simulink model "Microgrid_transition_model_111821_ben"  (R2020a)
settings: Solver=VariableStepAuto  StartTime=0.0  StopTime=16  MaxStep=1e-4  RelTol=1e-3
PreLoadFcn:
  | %run('FC_microgrid_param.m')
  | %load('gen_grid_init.mat')
InitFcn:
  | %load myisoModel_init;
  | run('FC_microgrid_param.m')
  | tic
  | run('CARTinitFcn.m')
  | %caseNo = 2;
  | 
  | %if (caseNo == 1)
  | %set_param(['Isolated_grid_paper_model_022521/SignalGen'], 'ActiveScenario', 'PStep222kW');
  | %else
  | %set_param(['Isolated_grid_paper_model_022521/SignalGen'], 'ActiveScenario', 'QStep222kVAr');
  | 
  | %end;
StopFcn:
  | toc
undefined symbols (not defined in the file): breakpoints1, breakpoints2, cc_kp, cp_table_data, ctrl, D1, Delta, DiscIntNeverNeededParam, DT, FC_BESS, FC_PV_FirstSolar, find_system, gcbh, libFC_BESS, libFC_PV, LowerLimit, magnitude, oversize, pll_ki, pll_kp, pq_ts, sps_rtmsupport, timer, Ts, ts, Ts_APC, Ts_Control, Ts_Power, UpperLimit
libraries: powerlib x152, powerlib_extras x100, simulink x95, powerlib_meascontrol x86, eePowerMeasurement x26, pi_ctrl x16, simulink_extras x12, sps_avr x7, spsDieselMotorModel x3, libFSArray x2, SignalEditorBlockLib x2, libLgBattery x1
(part 6 of 14)

== system Microgrid_transition_model_111821_ben/../Control/Speed & Pitch Control ==
  note: Current Regulator
  note: IL ref
  note: Note :
      | This control system is based on the report:
      | Dynamic Modeling of GE 1.5 and 3.6 Wind Turbine-Generators;
      | Prepared by: Nicholas W. Miller, William W. Price, Juan J. Sanchez-Gasca;
      | October 27, 2003, Version 3.0
      | GE-Power Systems Energy Consulting
      | Copyright 2002 General Electric Company, U.S.A.
      |
      | Another reference is:
      |
      | DYNAMIC MODELING OF GE 1.5 AND 3.6 MW WIND TURBINE GENERATORS
      | FOR STABILITY SIMULATIONS
      | Nicholas W. Miller, Juan J. Sanchez-Gasca, William W. Price Robert W. Delmerico
      | GE Power Systems GE Research
      | Schenectady, NY Niskayuna, NY
      |
      | 0-7803-7989-6/03/$17.00 02003 IEEE
  note: Speed Regulator
  note: Pitch Compensation
  note: Pitch Control
  wr : Inport
  Pmeas : Inport  Port=2
  IL : Inport  Port=3
  0-inf : Saturate  UpperLimit=inf  LowerLimit=0
  0-pitch_max : Saturate  UpperLimit=pitch_max  LowerLimit=0
  "0-pitch_max " : Saturate  UpperLimit=pitch_max  LowerLimit=0
  Constant2 : Constant
  Discrete PI Controller : Subsystem  DialogController=POWERSYS.PowerSysDialog  mask(Discrete PI Controller){Kp=Kp_speed, Ki=Ki_speed, Par_Limits=[1.1 0], Init=0, Ts=Ts}
      mask prompts: Kp "Proportional gain (Kp):"; Ki "Integral gain (Ki):"; Par_Limits "Output limits: [ Upper   Lower ]"; Init "Output initial value:"; Ts "Sample time:"
      mask help: This block implements a discrete PI controller.
      mask init:
      | UpperLimit=Par_Limits(1);
      | LowerLimit=Par_Limits(2);
      | power_initmask();
      mask Help: This block is part of a subset of blocks in the Extras library that does not have documentation associated with it, other than the block mask description.
      mask Display: disp('PI');
  Discrete PI Controller1 : Subsystem  DialogController=POWERSYS.PowerSysDialog  mask(Discrete PI Controller){Kp=Kp_compensation, Ki=Ki_compensation, Par_Limits=[pitch_max 0], Init=0, Ts=Ts}
      mask prompts: Kp "Proportional gain (Kp):"; Ki "Integral gain (Ki):"; Par_Limits "Output limits: [ Upper   Lower ]"; Init "Output initial value:"; Ts "Sample time:"
      mask help: This block implements a discrete PI controller.
      mask init:
      | UpperLimit=Par_Limits(1);
      | LowerLimit=Par_Limits(2);
      | power_initmask();
      mask Help: This block is part of a subset of blocks in the Extras library that does not have documentation associated with it, other than the block mask description.
      mask Display: disp('PI');
  Discrete PI Controller2 : Subsystem  DialogController=POWERSYS.PowerSysDialog  mask(Discrete PI Controller){Kp=Kp_boost_cur_reg, Ki=Ki_boost_cur_reg, Par_Limits=[1 0], Init=0.5, Ts=Ts}
      mask prompts: Kp "Proportional gain (Kp):"; Ki "Integral gain (Ki):"; Par_Limits "Output limits: [ Upper   Lower ]"; Init "Output initial value:"; Ts "Sample time:"
      mask help: This block implements a discrete PI controller.
      mask init:
      | UpperLimit=Par_Limits(1);
      | LowerLimit=Par_Limits(2);
      | power_initmask();
      mask Help: This block is part of a subset of blocks in the Extras library that does not have documentation associated with it, other than the block mask description.
      mask Display: disp('PI');
  First-Order Filter : powerlib_meascontrol/Filters/First-Order Filter  FilterType=Lowpass  Tc=Pitch_time_constant  Ts=Ts  Initialize=on  Vac_Init=[0.8 -25 60]*0  Vdc_Init=0  PlotResponse=off  FreqRange="[0,  200,  1]"
      settings: SourceProductBaseCode=MT,PS
  First-Order Filter1 : powerlib_meascontrol/Filters/First-Order Filter  FilterType=Lowpass  Tc=T_speed  Ts=Ts  Initialize=on  Vac_Init=[0, 0, 0]  Vdc_Init=1+init(1)/100  PlotResponse=off  FreqRange="[0,  200,  1]"
      settings: SourceProductBaseCode=MT,PS
  Gain2 : Gain  Gain=Kp_pitch  SaturateOnIntegerOverflow=on  OutDataTypeStr=Inherit: Same as input  ParamDataTypeStr=Inherit: Same as input
  Rate Limiter   1 : RateLimiter  RisingSlewLimit=pitch_rate  FallingSlewLimit=-pitch_rate
  Sum : Sum  Inputs=-+  SaturateOnIntegerOverflow=on
  Sum1 : Sum  Inputs=|+-
  Sum2 : Sum  Inputs=|+-  SaturateOnIntegerOverflow=on
  Sum3 : Sum  Inputs=|++
  Sum4 : Sum  Inputs=|+-
  Switch : Switch  Threshold=0.75
  Tracking Curve : Fcn  Expr=-0.5551*u(1)^2+1.183*u(1)+0.425
  pu_elec->pu_mec : Gain  Gain=Pnom/Pmec
  wref : Constant
  Duty_Cycle : Outport  VectorParamsAs1DForOutWhenUnconnected=off
  Pitch (deg) : Outport  Port=2  VectorParamsAs1DForOutWhenUnconnected=off
  wires:
  Discrete PI Controller2/1(Out) -> Duty_Cycle/1  "Duty cycle"
  IL/1 -> Sum4/2
  Sum4/1 -> Discrete PI Controller2/1(Error)
  Discrete PI Controller/1(Out) -> Sum4/1
  Tracking Curve/1 -> Switch/3
  First-Order Filter1/1 -> Sum/1, Sum1/2  "wref"
  Sum2/1 -> Discrete PI Controller1/1(Error)
  First-Order Filter/1 -> Pitch (deg)/1  "Pitch"
  Sum/1 -> Gain2/1
  "0-pitch_max "/1 -> First-Order Filter/1
  0-pitch_max/1 -> Sum3/1  "Pitch_contrl"
  Pmeas/1 -> 0-inf/1
  Discrete PI Controller1/1(Out) -> Sum3/2  "Pitch_comp"
  Gain2/1 -> 0-pitch_max/1
  Rate Limiter   1/1 -> "0-pitch_max "/1
  Sum3/1 -> Rate Limiter   1/1
  Constant2/1 -> Sum2/2  "Pref"
  Sum1/1 -> Discrete PI Controller/1(Error)
  Switch/1 -> First-Order Filter1/1
  wref/1 -> Switch/1
  pu_elec->pu_mec/1 -> Switch/2, Sum2/1, Tracking Curve/1  "Pmes"
  0-inf/1 -> pu_elec->pu_mec/1
  wr/1 -> Sum1/1, Sum/2  "wr"

== system Microgrid_transition_model_111821_ben/Defferable Load (0-446.25 kW)/Switches/Switches ABC0 ==
  P_ABC : Inport
  Demux : Demux  Outputs=3
      settings: DisplayOption=none
  Switch A : powerlib/Power Electronics/Ideal Switch  Ron=Ron_switch  Lon=0  IC=Status(1)  Rs=Rs_snubber  Cs=Cs_snubber  Measurements=off
      settings: AttributesFormatString=\n  SourceProductBaseCode=MT,PS
  Switch B : powerlib/Power Electronics/Ideal Switch  Ron=Ron_switch  Lon=0  IC=Status(1)  Rs=Rs_snubber  Cs=Cs_snubber  Measurements=off
      settings: AttributesFormatString=\n  SourceProductBaseCode=MT,PS
  Switch C : powerlib/Power Electronics/Ideal Switch  Ron=Ron_switch  Lon=0  IC=Status(1)  Rs=Rs_snubber  Cs=Cs_snubber  Measurements=off
      settings: AttributesFormatString=\n  SourceProductBaseCode=MT,PS
  A : PMIOPort  Side=Left
  B : PMIOPort  Port=2  Side=Left
  C : PMIOPort  Port=3  Side=Left
  "A " : PMIOPort  Port=4  Side=Right
  "B " : PMIOPort  Port=5  Side=Right
  "C " : PMIOPort  Port=6  Side=Right
  wires:
  P_ABC/1 -> Demux/1
  Demux/3 -> Switch C/1
  Demux/2 -> Switch B/1
  Demux/1 -> Switch A/1
  connections:
  Switch C/RConn1 -- "C "/RConn1
  Switch B/RConn1 -- "B "/RConn1
  Switch A/RConn1 -- "A "/RConn1
  C/RConn1 -- Switch C/LConn1
  B/RConn1 -- Switch B/LConn1
  A/RConn1 -- Switch A/LConn1

== system Microgrid_transition_model_111821_ben/Defferable Load (0-446.25 kW)/Switches/Switches ABC1 ==
  P_ABC : Inport
  Demux : Demux  Outputs=3
      settings: DisplayOption=none
  Switch A : powerlib/Power Electronics/Ideal Switch  Ron=Ron_switch  Lon=0  IC=Status(2)  Rs=Rs_snubber  Cs=Cs_snubber  Measurements=off
      settings: AttributesFormatString=\n  SourceProductBaseCode=MT,PS
  Switch B : powerlib/Power Electronics/Ideal Switch  Ron=Ron_switch  Lon=0  IC=Status(2)  Rs=Rs_snubber  Cs=Cs_snubber  Measurements=off
      settings: AttributesFormatString=\n  SourceProductBaseCode=MT,PS
  Switch C : powerlib/Power Electronics/Ideal Switch  Ron=Ron_switch  Lon=0  IC=Status(2)  Rs=Rs_snubber  Cs=Cs_snubber  Measurements=off
      settings: AttributesFormatString=\n  SourceProductBaseCode=MT,PS
  A : PMIOPort  Side=Left
  B : PMIOPort  Port=2  Side=Left
  C : PMIOPort  Port=3  Side=Left
  "A " : PMIOPort  Port=4  Side=Right
  "B " : PMIOPort  Port=5  Side=Right
  "C " : PMIOPort  Port=6  Side=Right
  wires:
  Demux/1 -> Switch A/1
  Demux/2 -> Switch B/1
  Demux/3 -> Switch C/1
  P_ABC/1 -> Demux/1
  connections:
  A/RConn1 -- Switch A/LConn1
  B/RConn1 -- Switch B/LConn1
  Switch A/RConn1 -- "A "/RConn1
  Switch B/RConn1 -- "B "/RConn1
  Switch C/RConn1 -- "C "/RConn1
  C/RConn1 -- Switch C/LConn1

== system Microgrid_transition_model_111821_ben/Defferable Load (0-446.25 kW)/Switches/Switches ABC2 ==
  P_ABC : Inport
  Demux : Demux  Outputs=3
      settings: DisplayOption=none
  Switch A : powerlib/Power Electronics/Ideal Switch  Ron=Ron_switch  Lon=0  IC=Status(3)  Rs=Rs_snubber  Cs=Cs_snubber  Measurements=off
      settings: AttributesFormatString=\n  SourceProductBaseCode=MT,PS
  Switch B : powerlib/Power Electronics/Ideal Switch  Ron=Ron_switch  Lon=0  IC=Status(3)  Rs=Rs_snubber  Cs=Cs_snubber  Measurements=off
      settings: AttributesFormatString=\n  SourceProductBaseCode=MT,PS
  Switch C : powerlib/Power Electronics/Ideal Switch  Ron=Ron_switch  Lon=0  IC=Status(3)  Rs=Rs_snubber  Cs=Cs_snubber  Measurements=off
      settings: AttributesFormatString=\n  SourceProductBaseCode=MT,PS
  A : PMIOPort  Side=Left
  B : PMIOPort  Port=2  Side=Left
  C : PMIOPort  Port=3  Side=Left
  "A " : PMIOPort  Port=4  Side=Right
  "B " : PMIOPort  Port=5  Side=Right
  "C " : PMIOPort  Port=6  Side=Right
  wires:
  P_ABC/1 -> Demux/1
  Demux/3 -> Switch C/1
  Demux/2 -> Switch B/1
  Demux/1 -> Switch A/1
  connections:
  Switch C/RConn1 -- "C "/RConn1
  Switch B/RConn1 -- "B "/RConn1
  Switch A/RConn1 -- "A "/RConn1
  A/RConn1 -- Switch A/LConn1
  B/RConn1 -- Switch B/LConn1
  C/RConn1 -- Switch C/LConn1

== system Microgrid_transition_model_111821_ben/Defferable Load (0-446.25 kW)/Switches/Switches ABC3 ==
  P_ABC : Inport
  Demux : Demux  Outputs=3
      settings: DisplayOption=none
  Switch A : powerlib/Power Electronics/Ideal Switch  Ron=Ron_switch  Lon=0  IC=Status(4)  Rs=Rs_snubber  Cs=Cs_snubber  Measurements=off
      settings: AttributesFormatString=\n  SourceProductBaseCode=MT,PS
  Switch B : powerlib/Power Electronics/Ideal Switch  Ron=Ron_switch  Lon=0  IC=Status(4)  Rs=Rs_snubber  Cs=Cs_snubber  Measurements=off
      settings: AttributesFormatString=\n  SourceProductBaseCode=MT,PS
  Switch C : powerlib/Power Electronics/Ideal Switch  Ron=Ron_switch  Lon=0  IC=Status(4)  Rs=Rs_snubber  Cs=Cs_snubber  Measurements=off
      settings: AttributesFormatString=\n  SourceProductBaseCode=MT,PS
  A : PMIOPort  Side=Left
  B : PMIOPort  Port=2  Side=Left
  C : PMIOPort  Port=3  Side=Left
  "A " : PMIOPort  Port=4  Side=Right
  "B " : PMIOPort  Port=5  Side=Right
  "C " : PMIOPort  Port=6  Side=Right
  wires:
  Demux/1 -> Switch A/1
  Demux/2 -> Switch B/1
  Demux/3 -> Switch C/1
  P_ABC/1 -> Demux/1
  connections:
  C/RConn1 -- Switch C/LConn1
  B/RConn1 -- Switch B/LConn1
  A/RConn1 -- Switch A/LConn1
  Switch A/RConn1 -- "A "/RConn1
  Switch B/RConn1 -- "B "/RConn1
  Switch C/RConn1 -- "C "/RConn1

== system Microgrid_transition_model_111821_ben/Defferable Load (0-446.25 kW)/Switches/Switches ABC4 ==
  P_ABC : Inport
  Demux : Demux  Outputs=3
      settings: DisplayOption=none
  Switch A : powerlib/Power Electronics/Ideal Switch  Ron=Ron_switch  Lon=0  IC=Status(5)  Rs=Rs_snubber  Cs=Cs_snubber  Measurements=off
      settings: AttributesFormatString=\n  SourceProductBaseCode=MT,PS
  Switch B : powerlib/Power Electronics/Ideal Switch  Ron=Ron_switch  Lon=0  IC=Status(5)  Rs=Rs_snubber  Cs=Cs_snubber  Measurements=off
      settings: AttributesFormatString=\n  SourceProductBaseCode=MT,PS
  Switch C : powerlib/Power Electronics/Ideal Switch  Ron=Ron_switch  Lon=0  IC=Status(5)  Rs=Rs_snubber  Cs=Cs_snubber  Measurements=off
      settings: AttributesFormatString=\n  SourceProductBaseCode=MT,PS
  A : PMIOPort  Side=Left
  B : PMIOPort  Port=2  Side=Left
  C : PMIOPort  Port=3  Side=Left
  "A " : PMIOPort  Port=4  Side=Right
  "B " : PMIOPort  Port=5  Side=Right
  "C " : PMIOPort  Port=6  Side=Right
  wires:
  P_ABC/1 -> Demux/1
  Demux/3 -> Switch C/1
  Demux/2 -> Switch B/1
  Demux/1 -> Switch A/1
  connections:
  Switch C/RConn1 -- "C "/RConn1
  Switch B/RConn1 -- "B "/RConn1
  Switch A/RConn1 -- "A "/RConn1
  A/RConn1 -- Switch A/LConn1
  B/RConn1 -- Switch B/LConn1
  C/RConn1 -- Switch C/LConn1

== system Microgrid_transition_model_111821_ben/Defferable Load (0-446.25 kW)/Switches/Switches ABC5 ==
  P_ABC : Inport
  Demux : Demux  Outputs=3
      settings: DisplayOption=none
  Switch A : powerlib/Power Electronics/Ideal Switch  Ron=Ron_switch  Lon=0  IC=Status(6)  Rs=Rs_snubber  Cs=Cs_snubber  Measurements=off
      settings: AttributesFormatString=\n  SourceProductBaseCode=MT,PS
  Switch B : powerlib/Power Electronics/Ideal Switch  Ron=Ron_switch  Lon=0  IC=Status(6)  Rs=Rs_snubber  Cs=Cs_snubber  Measurements=off
      settings: AttributesFormatString=\n  SourceProductBaseCode=MT,PS
  Switch C : powerlib/Power Electronics/Ideal Switch  Ron=Ron_switch  Lon=0  IC=Status(6)  Rs=Rs_snubber  Cs=Cs_snubber  Measurements=off
      settings: AttributesFormatString=\n  SourceProductBaseCode=MT,PS
  A : PMIOPort  Side=Left
  B : PMIOPort  Port=2  Side=Left
  C : PMIOPort  Port=3  Side=Left
  "A " : PMIOPort  Port=4  Side=Right
  "B " : PMIOPort  Port=5  Side=Right
  "C " : PMIOPort  Port=6  Side=Right
  wires:
  Demux/1 -> Switch A/1
  Demux/2 -> Switch B/1
  Demux/3 -> Switch C/1
  P_ABC/1 -> Demux/1
  connections:
  C/RConn1 -- Switch C/LConn1
  B/RConn1 -- Switch B/LConn1
  A/RConn1 -- Switch A/LConn1
  Switch A/RConn1 -- "A "/RConn1
  Switch B/RConn1 -- "B "/RConn1
  Switch C/RConn1 -- "C "/RConn1

== system Microgrid_transition_model_111821_ben/Defferable Load (0-446.25 kW)/Switches/Switches ABC6 ==
  P_ABC : Inport
  Demux : Demux  Outputs=3
      settings: DisplayOption=none
  Switch A : powerlib/Power Electronics/Ideal Switch  Ron=Ron_switch  Lon=0  IC=Status(7)  Rs=Rs_snubber  Cs=Cs_snubber  Measurements=off
      settings: AttributesFormatString=\n  SourceProductBaseCode=MT,PS
  Switch B : powerlib/Power Electronics/Ideal Switch  Ron=Ron_switch  Lon=0  IC=Status(7)  Rs=Rs_snubber  Cs=Cs_snubber  Measurements=off
      settings: AttributesFormatString=\n  SourceProductBaseCode=MT,PS
  Switch C : powerlib/Power Electronics/Ideal Switch  Ron=Ron_switch  Lon=0  IC=Status(7)  Rs=Rs_snubber  Cs=Cs_snubber  Measurements=off
      settings: AttributesFormatString=\n  SourceProductBaseCode=MT,PS
  A : PMIOPort  Side=Left
  B : PMIOPort  Port=2  Side=Left
  C : PMIOPort  Port=3  Side=Left
  "A " : PMIOPort  Port=4  Side=Right
  "B " : PMIOPort  Port=5  Side=Right
  "C " : PMIOPort  Port=6  Side=Right
  wires:
  P_ABC/1 -> Demux/1
  Demux/3 -> Switch C/1
  Demux/2 -> Switch B/1
  Demux/1 -> Switch A/1
  connections:
  Switch C/RConn1 -- "C "/RConn1
  Switch B/RConn1 -- "B "/RConn1
  Switch A/RConn1 -- "A "/RConn1
  A/RConn1 -- Switch A/LConn1
  B/RConn1 -- Switch B/LConn1
  C/RConn1 -- Switch C/LConn1

== system Microgrid_transition_model_111821_ben/Defferable Load (0-446.25 kW)/Switches/Switches ABC7 ==
  P_ABC : Inport
  Demux : Demux  Outputs=3
      settings: DisplayOption=none
  Switch A : powerlib/Power Electronics/Ideal Switch  Ron=Ron_switch  Lon=0  IC=Status(8)  Rs=Rs_snubber  Cs=Cs_snubber  Measurements=off
      settings: AttributesFormatString=\n  SourceProductBaseCode=MT,PS
  Switch B : powerlib/Power Electronics/Ideal Switch  Ron=Ron_switch  Lon=0  IC=Status(8)  Rs=Rs_snubber  Cs=Cs_snubber  Measurements=off
      settings: AttributesFormatString=\n  SourceProductBaseCode=MT,PS
  Switch C : powerlib/Power Electronics/Ideal Switch  Ron=Ron_switch  Lon=0  IC=Status(8)  Rs=Rs_snubber  Cs=Cs_snubber  Measurements=off
      settings: AttributesFormatString=\n  SourceProductBaseCode=MT,PS
  A : PMIOPort  Side=Left
  B : PMIOPort  Port=2  Side=Left
  C : PMIOPort  Port=3  Side=Left
  "A " : PMIOPort  Port=4  Side=Right
  "B " : PMIOPort  Port=5  Side=Right
  "C " : PMIOPort  Port=6  Side=Right
  wires:
  Demux/1 -> Switch A/1
  Demux/2 -> Switch B/1
  Demux/3 -> Switch C/1
  P_ABC/1 -> Demux/1
  connections:
  C/RConn1 -- Switch C/LConn1
  B/RConn1 -- Switch B/LConn1
  A/RConn1 -- Switch A/LConn1
  Switch A/RConn1 -- "A "/RConn1
  Switch B/RConn1 -- "B "/RConn1
  Switch C/RConn1 -- "C "/RConn1

== system Microgrid_transition_model_111821_ben/FC_BESS/SMAInverter/85_SMAControl ==
  Uabc : Inport
  Uabc_inv : Inport  Port=2
  Iabc : Inport  Port=3
  CB_status : Inport  Port=4
  Control : Inport  Port=5
  Bus Creator1 : BusCreator  Inputs=2
  Bus Creator5 : BusCreator  Inputs=1
  Bus Selector : BusSelector  OutputSignals=p_ref,q_ref,f_ref,v_ref,GF_mode
  InvControl : Subsystem  mask{Ts=Ts_Control, Unpp=400, Pn=1e6}
      mask prompts: Ts "Control sample time [s]"; Unpp "Nominal AC voltage [Vpp]"; Pn "Nominal Power [W]"
      mask init:
      | Unom = Unpp / sqrt(3);
      | Inom = Pn/3/Unom;
  Rate Transition{,1..2,4..7,9..10} (9 alike) : RateTransition  Integrity=off  OutPortSampleTime=Ts_Control
  Rate Transition3 : RateTransition  OutPortSampleTime=Ts
  Rate Transition8 : RateTransition  OutPortSampleTime=Ts
  Scope : Scope
  Step : Step  Time=3  Before=1  After=0  SampleTime=Ts
  Step1 : Step  Time=6.4  SampleTime=Ts
  Sum : Sum  Inputs=|++
  CtrlOut : Outport
  wires:
  Rate Transition4/1 -> InvControl/5(pref)
  Iabc/1 -> Rate Transition1/1
  Rate Transition2/1 -> InvControl/4(cb_stat)
  Rate Transition1/1 -> InvControl/3(Iabc)
  Rate Transition/1 -> InvControl/1(Uabc)
  Rate Transition8/1 -> Bus Creator5/1  "Close"
  Step/1 -> Sum/1
  InvControl/1(Uabc_ref) -> Rate Transition3/1
  Rate Transition3/1 -> Bus Creator1/1  "Uabc"
  Uabc/1 -> Rate Transition/1
  CB_status/1 -> Rate Transition2/1
  Bus Creator5/1 -> Bus Creator1/2  "ToCB"
  Bus Creator1/1 -> CtrlOut/1
  Bus Selector/1 -> Rate Transition4/1  "<p_ref>"
  Bus Selector/2 -> Rate Transition5/1  "<q_ref>"
  Bus Selector/3 -> Rate Transition6/1  "<f_ref>"
  Bus Selector/4 -> Rate Transition7/1  "<v_ref>"
  Bus Selector/5 -> Rate Transition9/1  "<GF_mode>"
  Rate Transition9/1 -> InvControl/9(GF_mode_en)
  Rate Transition7/1 -> InvControl/8(vref)
  Rate Transition5/1 -> InvControl/6(qref)
  Rate Transition6/1 -> InvControl/7(fref)
  Control/1 -> Bus Selector/1
  Uabc_inv/1 -> Rate Transition10/1
  Rate Transition10/1 -> InvControl/2(Uabc_inv)
  Step1/1 -> Sum/2
  Sum/1 -> Scope/1, Rate Transition8/1

== system Microgrid_transition_model_111821_ben/FC_BESS/SMAInverter/BESS Inverter ==
  ctrl : Inport
  Controlled Voltage Source : powerlib/Electrical Sources/Controlled Voltage Source  Initialize=on  Source_Type=AC  Amplitude=0  Phase=0  Frequency=0  Measurements=None
  Controlled Voltage Source1 : powerlib/Electrical Sources/Controlled Voltage Source  Initialize=on  Source_Type=AC  Amplitude=0  Phase=0  Frequency=0  Measurements=None
  Controlled Voltage Source2 : powerlib/Electrical Sources/Controlled Voltage Source  Initialize=on  Source_Type=AC  Amplitude=0  Phase=0  Frequency=0  Measurements=None
  Demux : Demux  Outputs=3
  A : PMIOPort  Side=Right
  N : PMIOPort  Port=2  Side=Left
  B : PMIOPort  Port=3  Side=Right
  C : PMIOPort  Port=4  Side=Right
  wires:
  ctrl/1 -> Demux/1
  Demux/3 -> Controlled Voltage Source2/1
  Demux/2 -> Controlled Voltage Source1/1
  Demux/1 -> Controlled Voltage Source/1
  connections:
  Controlled Voltage Source2/RConn1 -- C/RConn1
  Controlled Voltage Source1/RConn1 -- B/RConn1
  N/RConn1 -- Controlled Voltage Source1/LConn1 -- Controlled Voltage Source/LConn1 -- Controlled Voltage Source2/LConn1
  A/RConn1 -- Controlled Voltage Source/RConn1

== system Microgrid_transition_model_111821_ben/FC_BESS/SMAInverter/Subsystem ==
  GRI1 : powerlib/Measurements/Three-Phase V-I Measurement  VoltageMeasurement=phase-to-ground  SetLabelV=off  LabelV=Ugri  Vpu=off  VpuLL=off  CurrentMeasurement=yes  SetLabelI=off  LabelI=Igri  Ipu=off  Pbase=100e6  Vbase=500e3  OutputType=Complex  PhasorSimulation=off  PSBequivalent=0
  A : PMIOPort  Side=Left
  B : PMIOPort  Port=2  Side=Left
  a : PMIOPort  Port=3  Side=Right
  b : PMIOPort  Port=4  Side=Right
  C : PMIOPort  Port=5  Side=Left
  c : PMIOPort  Port=6  Side=Right
  tag scope: Igri=scoped, Ugri=scoped
  wires:
  GRI1/2 -> [Igri]
  GRI1/1 -> [Ugri]
  connections:
  GRI1/RConn1 -- a/RConn1
  GRI1/LConn1 -- A/RConn1
  GRI1/RConn2 -- b/RConn1
  GRI1/RConn3 -- c/RConn1
  GRI1/LConn2 -- B/RConn1
  GRI1/LConn3 -- C/RConn1

== system Microgrid_transition_model_111821_ben/FC_BESS/SMAInverter/Subsystem1 ==
  SmaINV : powerlib/Measurements/Three-Phase V-I Measurement  VoltageMeasurement=phase-to-ground  SetLabelV=off  LabelV=circuit_Usmainv  Vpu=off  VpuLL=off  CurrentMeasurement=yes  SetLabelI=off  LabelI=circuit_Ismainv  Ipu=off  Pbase=100e6  Vbase=500e3  OutputType=Complex  PhasorSimulation=off  PSBequivalent=0
  A : PMIOPort  Side=Left
  a : PMIOPort  Port=2  Side=Right
  B : PMIOPort  Port=3  Side=Left
  b : PMIOPort  Port=4  Side=Right
  C : PMIOPort  Port=5  Side=Left
  c : PMIOPort  Port=6  Side=Right
  tag scope: Iinv=scoped, Uinv=scoped
  wires:
  SmaINV/1 -> [Uinv]
  SmaINV/2 -> [Iinv]
  connections:
  SmaINV/RConn1 -- a/RConn1
  C/RConn1 -- SmaINV/LConn3
  SmaINV/LConn2 -- B/RConn1
  SmaINV/RConn2 -- b/RConn1
  SmaINV/RConn3 -- c/RConn1
  A/RConn1 -- SmaINV/LConn1

== system Microgrid_transition_model_111821_ben/FC_PV_FirstSolar/AllStringInverters/BESS Inverter ==
  ctrl : Inport
  Controlled Voltage Source : powerlib/Electrical Sources/Controlled Voltage Source  Initialize=on  Source_Type=AC  Amplitude=0  Phase=0  Frequency=0  Measurements=None
  Controlled Voltage Source1 : powerlib/Electrical Sources/Controlled Voltage Source  Initialize=on  Source_Type=AC  Amplitude=0  Phase=0  Frequency=0  Measurements=None
  Controlled Voltage Source2 : powerlib/Electrical Sources/Controlled Voltage Source  Initialize=on  Source_Type=AC  Amplitude=0  Phase=0  Frequency=0  Measurements=None
  Demux : Demux  Outputs=3
  A : PMIOPort  Side=Right
  N : PMIOPort  Port=2  Side=Left
  B : PMIOPort  Port=3  Side=Right
  C : PMIOPort  Port=4  Side=Right
  wires:
  Demux/1 -> Controlled Voltage Source/1
  Demux/2 -> Controlled Voltage Source1/1
  Demux/3 -> Controlled Voltage Source2/1
  ctrl/1 -> Demux/1
  connections:
  A/RConn1 -- Controlled Voltage Source/RConn1
  Controlled Voltage Source2/LConn1 -- Controlled Voltage Source/LConn1 -- Controlled Voltage Source1/LConn1 -- N/RConn1
  Controlled Voltage Source1/RConn1 -- B/RConn1
  Controlled Voltage Source2/RConn1 -- C/RConn1

== system Microgrid_transition_model_111821_ben/FC_PV_FirstSolar/AllStringInverters/PV_Control ==
  Uabc : Inport
  Uabc_inv : Inport  Port=2
  Iabc : Inport  Port=3
  CB_status : Inport  Port=4
  Control : Inport  Port=5
  Ppv : Inport  Port=6
  Bus Creator1 : BusCreator  Inputs=2
  Bus Creator5 : BusCreator  Inputs=1
  Bus Selector : BusSelector  OutputSignals=p_ref,q_ref,f_ref,v_ref,GF_mode
  InvControl : Subsystem  mask{Ts=Ts_Control, Unpp=600, Pn=430e3}
      mask prompts: Ts "Control sample time [s]"; Unpp "Nominal AC voltage [Vpp]"; Pn "Nominal Power [W]"
      mask init:
      | Unom = Unpp / sqrt(3);
      | Inom = Pn/3/Unom;
  Min : MinMax  Inputs=2
  Rate Transition{,1..2,4..7,9..10} (9 alike) : RateTransition  Integrity=off  OutPortSampleTime=Ts_Control
  Rate Transition3 : RateTransition  OutPortSampleTime=Ts
  Rate Transition8 : RateTransition  OutPortSampleTime=Ts
  Step : Step  Time=0.5  SampleTime=0
  Step1 : Step  Time=99  After=-1  SampleTime=0
  Sum : Sum  Inputs=|++
  CtrlOut : Outport
  wires:
  Rate Transition10/1 -> InvControl/2(Uabc_inv)
  Uabc_inv/1 -> Rate Transition10/1
  Control/1 -> Bus Selector/1
  Rate Transition6/1 -> InvControl/7(fref)
  Rate Transition5/1 -> InvControl/6(qref)
  Rate Transition7/1 -> InvControl/8(vref)
  Rate Transition9/1 -> InvControl/9(GF_mode_en)
  Bus Selector/5 -> Rate Transition9/1  "<GF_mode>"
  Bus Selector/4 -> Rate Transition7/1  "<v_ref>"
  Bus Selector/3 -> Rate Transition6/1  "<f_ref>"
  Bus Selector/2 -> Rate Transition5/1  "<q_ref>"
  Bus Selector/1 -> Min/1  "<p_ref>"
  Bus Creator1/1 -> CtrlOut/1
  Bus Creator5/1 -> Bus Creator1/2  "ToCB"
  CB_status/1 -> Rate Transition2/1
  Uabc/1 -> Rate Transition/1
  Rate Transition3/1 -> Bus Creator1/1  "Uabc"
  InvControl/1(Uabc_ref) -> Rate Transition3/1
  Step/1 -> Sum/1
  Rate Transition8/1 -> Bus Creator5/1  "Close"
  Rate Transition/1 -> InvControl/1(Uabc)
  Rate Transition1/1 -> InvControl/3(Iabc)
  Rate Transition2/1 -> InvControl/4(cb_stat)
  Iabc/1 -> Rate Transition1/1
  Rate Transition4/1 -> InvControl/5(pref)
  Ppv/1 -> Min/2
  Min/1 -> Rate Transition4/1
  Step1/1 -> Sum/2
  Sum/1 -> Rate Transition8/1

== system Microgrid_transition_model_111821_ben/FC_PV_FirstSolar/AllStringInverters/Subsystem1 ==
  SmaINV : powerlib/Measurements/Three-Phase V-I Measurement  VoltageMeasurement=phase-to-ground  SetLabelV=off  LabelV=circuit_Usmainv  Vpu=off  VpuLL=off  CurrentMeasurement=yes  SetLabelI=off  LabelI=circuit_Ismainv  Ipu=off  Pbase=100e6  Vbase=500e3  OutputType=Complex  PhasorSimulation=off  PSBequivalent=0
  A : PMIOPort  Side=Left
  a : PMIOPort  Port=2  Side=Right
  B : PMIOPort  Port=3  Side=Left
  b : PMIOPort  Port=4  Side=Right
  C : PMIOPort  Port=5  Side=Left
  c : PMIOPort  Port=6  Side=Right
  tag scope: Iinv=scoped, Uinv=scoped
  wires:
  SmaINV/1 -> [Uinv]
  SmaINV/2 -> [Iinv]
  connections:
  SmaINV/RConn1 -- a/RConn1
  C/RConn1 -- SmaINV/LConn3
  SmaINV/LConn2 -- B/RConn1
  SmaINV/RConn2 -- b/RConn1
  SmaINV/RConn3 -- c/RConn1
  A/RConn1 -- SmaINV/LConn1

== system Microgrid_transition_model_111821_ben/FC_PV_FirstSolar/AllStringInverters/Subsystem2 ==
  GRI1 : powerlib/Measurements/Three-Phase V-I Measurement  VoltageMeasurement=phase-to-ground  SetLabelV=off  LabelV=Ugri  Vpu=off  VpuLL=off  CurrentMeasurement=yes  SetLabelI=off  LabelI=Igri  Ipu=off  Pbase=100e6  Vbase=500e3  OutputType=Complex  PhasorSimulation=off  PSBequivalent=0
  A : PMIOPort  Side=Left
  B : PMIOPort  Port=2  Side=Left
  a : PMIOPort  Port=3  Side=Right
  b : PMIOPort  Port=4  Side=Right
  C : PMIOPort  Port=5  Side=Left
  c : PMIOPort  Port=6  Side=Right
  tag scope: Igri=scoped, Ugri=scoped
  wires:
  GRI1/1 -> [Ugri]
  GRI1/2 -> [Igri]
  connections:
  GRI1/LConn3 -- C/RConn1
  GRI1/LConn2 -- B/RConn1
  GRI1/RConn3 -- c/RConn1
  GRI1/RConn2 -- b/RConn1
  GRI1/LConn1 -- A/RConn1
  GRI1/RConn1 -- a/RConn1

== system Microgrid_transition_model_111821_ben/Grid Feeder Protective Relay/CS Modified PLL/Controller ==
  note: Pierre Giroux, Gilbert Sybille
      | Power System Simulation Laboratory
      | IREQ, Hydro-Quebc
  note: Discrete PID Controller
  Error : Inport
  Discrete Derivative : simulink/Discrete/Discrete Derivative  gainval=1.0  ICPrevScaledInput=0.0  OutMin=[]  OutMax=[]  OutDataType=sfix(16)  OutScaling=2^-10  DoSatur=off
  Discrete-Time Integrator : DiscreteIntegrator  InitialCondition=Init  SampleTime=Ts  LimitOutput=on  UpperSaturationLimit=UpperLimit  LowerSaturationLimit=LowerLimit  ICPrevOutput=DiscIntNeverNeededParam  ICPrevScaledInput=DiscIntNeverNeededParam
  Kp4 : Gain  Gain=Kp  SaturateOnIntegerOverflow=on  OutDataTypeStr=Inherit: Same as input  ParamDataTypeStr=Inherit: Same as input
  Kp5 : Gain  Gain=Ki  SaturateOnIntegerOverflow=on  OutDataTypeStr=Inherit: Same as input  ParamDataTypeStr=Inherit: Same as input
  Kp6 : Gain  Gain=Kd  SaturateOnIntegerOverflow=on  OutDataTypeStr=Inherit: Same as input  ParamDataTypeStr=Inherit: Same as input
  Saturation2 : Saturate  UpperLimit=UpperLimit  LowerLimit=LowerLimit
  Sum6 : Sum  Inputs=+++  InputSameDT=on  SaturateOnIntegerOverflow=on  OutDataTypeStr=Inherit: Same as first input
  Zero-Order Hold : ZeroOrderHold  SampleTime=Ts
  Out : Outport  InitialOutput=0
  wires:
  Error/1 -> Kp4/1, Kp5/1, Kp6/1
  Sum6/1 -> Saturation2/1
  Kp5/1 -> Discrete-Time Integrator/1
  Kp6/1 -> Zero-Order Hold/1
  Kp4/1 -> Sum6/1
  Discrete-Time Integrator/1 -> Sum6/2
  Discrete Derivative/1 -> Sum6/3
  Saturation2/1 -> Out/1
  Zero-Order Hold/1 -> Discrete Derivative/1

== system Microgrid_transition_model_111821_ben/Grid Feeder Protective Relay/CS Modified PLL/VCO ==
  w : Inport
  Compare To Constant : simulink/Logic and Bit Operations/Compare To Constant  relop=>=  const=pi  OutDataTypeStr=uint8
  Gain : Gain  Gain=2*pi  OutDataTypeStr=double
  Gain2 : Gain  Gain=Ts  SaturateOnIntegerOverflow=on  OutDataTypeStr=Inherit: Same as input  ParamDataTypeStr=Inherit: Same as input
  Sum : Sum  Inputs=-++
  Unit Delay1 : UnitDelay  SampleTime=-1  HasFrameUpgradeWarning=on
  theta : Outport
  wires:
  w/1 -> Gain2/1
  Gain/1 -> Sum/1
  Compare To Constant/1 -> Gain/1
  Unit Delay1/1 -> Compare To Constant/1, Sum/3, theta/1  "wt"
  Gain2/1 -> Sum/2
  Sum/1 -> Unit Delay1/1

== system Microgrid_transition_model_111821_ben/Grid Feeder Protective Relay/CS Modified PLL1/Controller ==
  note: Pierre Giroux, Gilbert Sybille
      | Power System Simulation Laboratory
      | IREQ, Hydro-Quebc
  note: Discrete PID Controller
  Error : Inport
  Discrete Derivative : simulink/Discrete/Discrete Derivative  gainval=1.0  ICPrevScaledInput=0.0  OutMin=[]  OutMax=[]  OutDataType=sfix(16)  OutScaling=2^-10  DoSatur=off
  Discrete-Time Integrator : DiscreteIntegrator  InitialCondition=Init  SampleTime=Ts  LimitOutput=on  UpperSaturationLimit=UpperLimit  LowerSaturationLimit=LowerLimit  ICPrevOutput=DiscIntNeverNeededParam  ICPrevScaledInput=DiscIntNeverNeededParam
  Kp4 : Gain  Gain=Kp  SaturateOnIntegerOverflow=on  OutDataTypeStr=Inherit: Same as input  ParamDataTypeStr=Inherit: Same as input
  Kp5 : Gain  Gain=Ki  SaturateOnIntegerOverflow=on  OutDataTypeStr=Inherit: Same as input  ParamDataTypeStr=Inherit: Same as input
  Kp6 : Gain  Gain=Kd  SaturateOnIntegerOverflow=on  OutDataTypeStr=Inherit: Same as input  ParamDataTypeStr=Inherit: Same as input
  Saturation2 : Saturate  UpperLimit=UpperLimit  LowerLimit=LowerLimit
  Sum6 : Sum  Inputs=+++  InputSameDT=on  SaturateOnIntegerOverflow=on  OutDataTypeStr=Inherit: Same as first input
  Zero-Order Hold : ZeroOrderHold  SampleTime=Ts
  Out : Outport  InitialOutput=0
  wires:
  Error/1 -> Kp4/1, Kp5/1, Kp6/1
  Sum6/1 -> Saturation2/1
  Kp5/1 -> Discrete-Time Integrator/1
  Kp6/1 -> Zero-Order Hold/1
  Kp4/1 -> Sum6/1
  Discrete-Time Integrator/1 -> Sum6/2
  Discrete Derivative/1 -> Sum6/3
  Saturation2/1 -> Out/1
  Zero-Order Hold/1 -> Discrete Derivative/1

== system Microgrid_transition_model_111821_ben/Grid Feeder Protective Relay/CS Modified PLL1/VCO ==
  w : Inport
  Compare To Constant : simulink/Logic and Bit Operations/Compare To Constant  relop=>=  const=pi  OutDataTypeStr=uint8
  Gain : Gain  Gain=2*pi  OutDataTypeStr=double
  Gain2 : Gain  Gain=Ts  SaturateOnIntegerOverflow=on  OutDataTypeStr=Inherit: Same as input  ParamDataTypeStr=Inherit: Same as input
  Sum : Sum  Inputs=-++
  Unit Delay1 : UnitDelay  SampleTime=-1  HasFrameUpgradeWarning=on
  theta : Outport
  wires:
  w/1 -> Gain2/1
  Gain/1 -> Sum/1
  Compare To Constant/1 -> Gain/1
  Unit Delay1/1 -> Compare To Constant/1, Sum/3, theta/1  "wt"
  Gain2/1 -> Sum/2
  Sum/1 -> Unit Delay1/1

== system Microgrid_transition_model_111821_ben/Grid Feeder Protective Relay/R25 - Sync Check v0.1/Freq_Comparator ==
  note: This block compares the frequency at the circuit breaker terminals
      | * if the difference is less than threshold dF_threshold, then outputs 1
  f_grid : Inport
  f_gen : Inport  Port=2
  dF_threshold : Inport  Port=3
  Fcn2 : Fcn  Expr=abs(u(2)-u(1)) <= u(3)
  Mux1 : Mux  Inputs=3
  Sum : Sum  Inputs=+-
  Locked : Outport
  dF : Outport  Port=2
  wires:
  Sum/1 -> dF/1
  f_grid/1 -> Mux1/1, Sum/2
  f_gen/1 -> Mux1/2, Sum/1
  dF_threshold/1 -> Mux1/3
  Fcn2/1 -> Locked/1
  Mux1/1 -> Fcn2/1

== system Microgrid_transition_model_111821_ben/Grid Feeder Protective Relay/R25 - Sync Check v0.1/Phase_Comparator ==
  note: This block compares the angle (phase A only) at the circuit breaker terminals
      | * if the difference is less than threshold angle_threshold, then outputs 1
  wt_grid : Inport
  wt_gen : Inport  Port=2
  angle_threshold : Inport  Port=3
  Abs : Abs
  Fcn1 : Fcn  Expr=u(1) <= u(2)  SampleTime=Ts
  Mux1 : Mux  Inputs=2
  Radians to Degrees : simulink_extras/Transformations/Radians to Degrees
  Scope : Scope
  Sum1 : Sum  Inputs=|-+
  WrapPi : Subsystem
  Locked : Outport
  dWt : Outport  Port=2
  wires:
  WrapPi/1(Out1) -> Abs/1, dWt/1
  Sum1/1 -> WrapPi/1(In1)
  wt_grid/1 -> Sum1/1
  wt_gen/1 -> Sum1/2
  Radians to Degrees/1 -> Scope/1, Mux1/1  "R2D"
  Mux1/1 -> Fcn1/1
  angle_threshold/1 -> Mux1/2
  Fcn1/1 -> Locked/1  "bool"
  Abs/1 -> Radians to Degrees/1  "diff"

== system Microgrid_transition_model_111821_ben/Grid Feeder Protective Relay/R25 - Sync Check v0.1/Voltage_Comparator ==
  note: This block compares the voltage at the circuit breaker terminals
      | * if the difference is less than threshold, then outputs 1
  note: dV_threshold% of the nominal VRMSLL
  V_bus : Inport
  V_line : Inport  Port=2
  dV_threshold : Inport  Port=3
  Fcn2 : Fcn  Expr=abs(u(2)-u(1)) <= u(3)
  Mux1 : Mux  Inputs=3
  Sum : Sum  Inputs=+-
  Locked : Outport
  dV : Outport  Port=2
  wires:
  Sum/1 -> dV/1
  dV_threshold/1 -> Mux1/3  "[%]"
  V_bus/1 -> Sum/2, Mux1/1
  V_line/1 -> Mux1/2, Sum/1
  Fcn2/1 -> Locked/1  "thshld"
  Mux1/1 -> Fcn2/1

== system Microgrid_transition_model_111821_ben/Grid Feeder Protective Relay1/CS Modified PLL/Controller ==
  note: Discrete PID Controller
  note: Pierre Giroux, Gilbert Sybille
      | Power System Simulation Laboratory
      | IREQ, Hydro-Quebc
  Error : Inport
  Discrete Derivative : simulink/Discrete/Discrete Derivative  gainval=1.0  ICPrevScaledInput=0.0  OutMin=[]  OutMax=[]  OutDataType=sfix(16)  OutScaling=2^-10  DoSatur=off
  Discrete-Time Integrator : DiscreteIntegrator  InitialCondition=Init  SampleTime=Ts  LimitOutput=on  UpperSaturationLimit=UpperLimit  LowerSaturationLimit=LowerLimit  ICPrevOutput=DiscIntNeverNeededParam  ICPrevScaledInput=DiscIntNeverNeededParam
  Kp4 : Gain  Gain=Kp  SaturateOnIntegerOverflow=on  OutDataTypeStr=Inherit: Same as input  ParamDataTypeStr=Inherit: Same as input
  Kp5 : Gain  Gain=Ki  SaturateOnIntegerOverflow=on  OutDataTypeStr=Inherit: Same as input  ParamDataTypeStr=Inherit: Same as input
  Kp6 : Gain  Gain=Kd  SaturateOnIntegerOverflow=on  OutDataTypeStr=Inherit: Same as input  ParamDataTypeStr=Inherit: Same as input
  Saturation2 : Saturate  UpperLimit=UpperLimit  LowerLimit=LowerLimit
  Sum6 : Sum  Inputs=+++  InputSameDT=on  SaturateOnIntegerOverflow=on  OutDataTypeStr=Inherit: Same as first input
  Zero-Order Hold : ZeroOrderHold  SampleTime=Ts
  Out : Outport  InitialOutput=0
  wires:
  Zero-Order Hold/1 -> Discrete Derivative/1
  Saturation2/1 -> Out/1
  Discrete Derivative/1 -> Sum6/3
  Discrete-Time Integrator/1 -> Sum6/2
  Kp4/1 -> Sum6/1
  Kp6/1 -> Zero-Order Hold/1
  Kp5/1 -> Discrete-Time Integrator/1
  Sum6/1 -> Saturation2/1
  Error/1 -> Kp6/1, Kp5/1, Kp4/1

== system Microgrid_transition_model_111821_ben/Grid Feeder Protective Relay1/CS Modified PLL/VCO ==
  w : Inport
  Compare To Constant : simulink/Logic and Bit Operations/Compare To Constant  relop=>=  const=pi  OutDataTypeStr=uint8
  Gain : Gain  Gain=2*pi  OutDataTypeStr=double
  Gain2 : Gain  Gain=Ts  SaturateOnIntegerOverflow=on  OutDataTypeStr=Inherit: Same as input  ParamDataTypeStr=Inherit: Same as input
  Sum : Sum  Inputs=-++
  Unit Delay1 : UnitDelay  SampleTime=-1  HasFrameUpgradeWarning=on
  theta : Outport
  wires:
  Sum/1 -> Unit Delay1/1
  Gain2/1 -> Sum/2
  Unit Delay1/1 -> theta/1, Sum/3, Compare To Constant/1  "wt"
  Compare To Constant/1 -> Gain/1
  Gain/1 -> Sum/1
  w/1 -> Gain2/1

== system Microgrid_transition_model_111821_ben/Grid Feeder Protective Relay1/CS Modified PLL1/Controller ==
  note: Discrete PID Controller
  note: Pierre Giroux, Gilbert Sybille
      | Power System Simulation Laboratory
      | IREQ, Hydro-Quebc
  Error : Inport
  Discrete Derivative : simulink/Discrete/Discrete Derivative  gainval=1.0  ICPrevScaledInput=0.0  OutMin=[]  OutMax=[]  OutDataType=sfix(16)  OutScaling=2^-10  DoSatur=off
  Discrete-Time Integrator : DiscreteIntegrator  InitialCondition=Init  SampleTime=Ts  LimitOutput=on  UpperSaturationLimit=UpperLimit  LowerSaturationLimit=LowerLimit  ICPrevOutput=DiscIntNeverNeededParam  ICPrevScaledInput=DiscIntNeverNeededParam
  Kp4 : Gain  Gain=Kp  SaturateOnIntegerOverflow=on  OutDataTypeStr=Inherit: Same as input  ParamDataTypeStr=Inherit: Same as input
  Kp5 : Gain  Gain=Ki  SaturateOnIntegerOverflow=on  OutDataTypeStr=Inherit: Same as input  ParamDataTypeStr=Inherit: Same as input
  Kp6 : Gain  Gain=Kd  SaturateOnIntegerOverflow=on  OutDataTypeStr=Inherit: Same as input  ParamDataTypeStr=Inherit: Same as input
  Saturation2 : Saturate  UpperLimit=UpperLimit  LowerLimit=LowerLimit
  Sum6 : Sum  Inputs=+++  InputSameDT=on  SaturateOnIntegerOverflow=on  OutDataTypeStr=Inherit: Same as first input
  Zero-Order Hold : ZeroOrderHold  SampleTime=Ts
  Out : Outport  InitialOutput=0
  wires:
  Zero-Order Hold/1 -> Discrete Derivative/1
  Saturation2/1 -> Out/1
  Discrete Derivative/1 -> Sum6/3
  Discrete-Time Integrator/1 -> Sum6/2
  Kp4/1 -> Sum6/1
  Kp6/1 -> Zero-Order Hold/1
  Kp5/1 -> Discrete-Time Integrator/1
  Sum6/1 -> Saturation2/1
  Error/1 -> Kp6/1, Kp5/1, Kp4/1

== system Microgrid_transition_model_111821_ben/Grid Feeder Protective Relay1/CS Modified PLL1/VCO ==
  w : Inport
  Compare To Constant : simulink/Logic and Bit Operations/Compare To Constant  relop=>=  const=pi  OutDataTypeStr=uint8
  Gain : Gain  Gain=2*pi  OutDataTypeStr=double
  Gain2 : Gain  Gain=Ts  SaturateOnIntegerOverflow=on  OutDataTypeStr=Inherit: Same as input  ParamDataTypeStr=Inherit: Same as input
  Sum : Sum  Inputs=-++
  Unit Delay1 : UnitDelay  SampleTime=-1  HasFrameUpgradeWarning=on
  theta : Outport
  wires:
  Sum/1 -> Unit Delay1/1
  Gain2/1 -> Sum/2
  Unit Delay1/1 -> theta/1, Sum/3, Compare To Constant/1  "wt"
  Compare To Constant/1 -> Gain/1
  Gain/1 -> Sum/1
  w/1 -> Gain2/1

== system Microgrid_transition_model_111821_ben/Grid Feeder Protective Relay1/R25 - Sync Check v0.1/Freq_Comparator ==
  note: This block compares the frequency at the circuit breaker terminals
      | * if the difference is less than threshold dF_threshold, then outputs 1
  f_grid : Inport
  f_gen : Inport  Port=2
  dF_threshold : Inport  Port=3
  Fcn2 : Fcn  Expr=abs(u(2)-u(1)) <= u(3)
  Mux1 : Mux  Inputs=3
  Sum : Sum  Inputs=+-
  Locked : Outport
  dF : Outport  Port=2
  wires:
  Mux1/1 -> Fcn2/1
  Fcn2/1 -> Locked/1
  dF_threshold/1 -> Mux1/3
  f_gen/1 -> Sum/1, Mux1/2
  f_grid/1 -> Sum/2, Mux1/1
  Sum/1 -> dF/1

== system Microgrid_transition_model_111821_ben/Grid Feeder Protective Relay1/R25 - Sync Check v0.1/Phase_Comparator ==
  note: This block compares the angle (phase A only) at the circuit breaker terminals
      | * if the difference is less than threshold angle_threshold, then outputs 1
  wt_grid : Inport
  wt_gen : Inport  Port=2
  angle_threshold : Inport  Port=3
  Abs : Abs
  Fcn1 : Fcn  Expr=u(1) <= u(2)  SampleTime=Ts
  Mux1 : Mux  Inputs=2
  Radians to Degrees : simulink_extras/Transformations/Radians to Degrees
  Scope : Scope
  Sum1 : Sum  Inputs=|-+
  WrapPi : Subsystem
  Locked : Outport
  dWt : Outport  Port=2
  wires:
  Abs/1 -> Radians to Degrees/1  "diff"
  Fcn1/1 -> Locked/1  "bool"
  angle_threshold/1 -> Mux1/2
  Mux1/1 -> Fcn1/1
  Radians to Degrees/1 -> Scope/1, Mux1/1  "R2D"
  wt_gen/1 -> Sum1/2
  wt_grid/1 -> Sum1/1
  Sum1/1 -> WrapPi/1(In1)
  WrapPi/1(Out1) -> dWt/1, Abs/1

== system Microgrid_transition_model_111821_ben/Grid Feeder Protective Relay1/R25 - Sync Check v0.1/Voltage_Comparator ==
  note: dV_threshold% of the nominal VRMSLL
  note: This block compares the voltage at the circuit breaker terminals
      | * if the difference is less than threshold, then outputs 1
  V_bus : Inport
  V_line : Inport  Port=2
  dV_threshold : Inport  Port=3
  Fcn2 : Fcn  Expr=abs(u(2)-u(1)) <= u(3)
  Mux1 : Mux  Inputs=3
  Sum : Sum  Inputs=+-
  Locked : Outport
  dV : Outport  Port=2
  wires:
  Mux1/1 -> Fcn2/1
  Fcn2/1 -> Locked/1  "thshld"
  V_line/1 -> Sum/1, Mux1/2
  V_bus/1 -> Mux1/1, Sum/2
  dV_threshold/1 -> Mux1/3  "[%]"
  Sum/1 -> dV/1

== system Microgrid_transition_model_111821_ben/MODEL STABILIZER/AllStringInverters/BESS Inverter ==
  ctrl : Inport
  Controlled Voltage Source : powerlib/Electrical Sources/Controlled Voltage Source  Initialize=on  Source_Type=AC  Amplitude=0  Phase=0  Frequency=0  Measurements=None
  Controlled Voltage Source1 : powerlib/Electrical Sources/Controlled Voltage Source  Initialize=on  Source_Type=AC  Amplitude=0  Phase=0  Frequency=0  Measurements=None
  Controlled Voltage Source2 : powerlib/Electrical Sources/Controlled Voltage Source  Initialize=on  Source_Type=AC  Amplitude=0  Phase=0  Frequency=0  Measurements=None
  Demux : Demux  Outputs=3
  A : PMIOPort  Side=Right
  N : PMIOPort  Port=2  Side=Left
  B : PMIOPort  Port=3  Side=Right
  C : PMIOPort  Port=4  Side=Right
  wires:
  Demux/1 -> Controlled Voltage Source/1
  Demux/2 -> Controlled Voltage Source1/1
  Demux/3 -> Controlled Voltage Source2/1
  ctrl/1 -> Demux/1
  connections:
  A/RConn1 -- Controlled Voltage Source/RConn1
  Controlled Voltage Source2/LConn1 -- Controlled Voltage Source/LConn1 -- Controlled Voltage Source1/LConn1 -- N/RConn1
  Controlled Voltage Source1/RConn1 -- B/RConn1
  Controlled Voltage Source2/RConn1 -- C/RConn1

== system Microgrid_transition_model_111821_ben/MODEL STABILIZER/AllStringInverters/Stab_control ==
  Uabc : Inport
  Uabc_inv : Inport  Port=2
  Iabc : Inport  Port=3
  CB_status : Inport  Port=4
  Control : Inport  Port=5
  Bus Creator1 : BusCreator  Inputs=2
  Bus Creator5 : BusCreator  Inputs=1
  Bus Selector : BusSelector  OutputSignals=p_ref,q_ref,f_ref,v_ref,GF_mode
  InvControl : Subsystem  mask{Ts=Ts_Control, Unpp=600, Pn=100e3}
      mask prompts: Ts "Control sample time [s]"; Unpp "Nominal AC voltage [Vpp]"; Pn "Nominal Power [W]"
      mask init:
      | Unom = Unpp / sqrt(3);
      | Inom = Pn/3/Unom;
  Rate Transition{,1..2,4..7,9..10} (9 alike) : RateTransition  Integrity=off  OutPortSampleTime=Ts_Control
  Rate Transition3 : RateTransition  OutPortSampleTime=Ts
  Rate Transition8 : RateTransition  OutPortSampleTime=Ts
  Step1 : Step  Time=3  SampleTime=0
  Step2 : Step  Time=6.4  After=-1  SampleTime=0
  Sum : Sum  Inputs=|++
  CtrlOut : Outport
  wires:
  Sum/1 -> Rate Transition8/1
  Rate Transition10/1 -> InvControl/2(Uabc_inv)
  Uabc_inv/1 -> Rate Transition10/1
  Control/1 -> Bus Selector/1
  Rate Transition6/1 -> InvControl/7(fref)
  Rate Transition5/1 -> InvControl/6(qref)
  Rate Transition7/1 -> InvControl/8(vref)
  Rate Transition9/1 -> InvControl/9(GF_mode_en)
  Bus Selector/5 -> Rate Transition9/1  "<GF_mode>"
  Bus Selector/4 -> Rate Transition7/1  "<v_ref>"
  Bus Selector/3 -> Rate Transition6/1  "<f_ref>"
  Bus Selector/2 -> Rate Transition5/1  "<q_ref>"
  Bus Selector/1 -> Rate Transition4/1  "<p_ref>"
  Bus Creator1/1 -> CtrlOut/1
  Bus Creator5/1 -> Bus Creator1/2  "ToCB"
  CB_status/1 -> Rate Transition2/1
  Uabc/1 -> Rate Transition/1
  Rate Transition3/1 -> Bus Creator1/1  "Uabc"
  InvControl/1(Uabc_ref) -> Rate Transition3/1
  Rate Transition8/1 -> Bus Creator5/1  "Close"
  Rate Transition/1 -> InvControl/1(Uabc)
  Rate Transition1/1 -> InvControl/3(Iabc)
  Rate Transition2/1 -> InvControl/4(cb_stat)
  Iabc/1 -> Rate Transition1/1
  Rate Transition4/1 -> InvControl/5(pref)
  Step1/1 -> Sum/1
  Step2/1 -> Sum/2

== system Microgrid_transition_model_111821_ben/MODEL STABILIZER/AllStringInverters/Subsystem1 ==
  SmaINV : powerlib/Measurements/Three-Phase V-I Measurement  VoltageMeasurement=phase-to-ground  SetLabelV=off  LabelV=circuit_Usmainv  Vpu=off  VpuLL=off  CurrentMeasurement=yes  SetLabelI=off  LabelI=circuit_Ismainv  Ipu=off  Pbase=100e6  Vbase=500e3  OutputType=Complex  PhasorSimulation=off  PSBequivalent=0
  A : PMIOPort  Side=Left
  a : PMIOPort  Port=2  Side=Right
  B : PMIOPort  Port=3  Side=Left
  b : PMIOPort  Port=4  Side=Right
  C : PMIOPort  Port=5  Side=Left
  c : PMIOPort  Port=6  Side=Right
  tag scope: Iinv=scoped, Uinv=scoped
  wires:
  SmaINV/1 -> [Uinv]
  SmaINV/2 -> [Iinv]
  connections:
  SmaINV/RConn1 -- a/RConn1
  C/RConn1 -- SmaINV/LConn3
  SmaINV/LConn2 -- B/RConn1
  SmaINV/RConn2 -- b/RConn1
  SmaINV/RConn3 -- c/RConn1
  A/RConn1 -- SmaINV/LConn1

== system Microgrid_transition_model_111821_ben/MODEL STABILIZER/AllStringInverters/Subsystem2 ==
  GRI1 : powerlib/Measurements/Three-Phase V-I Measurement  VoltageMeasurement=phase-to-ground  SetLabelV=off  LabelV=Ugri  Vpu=off  VpuLL=off  CurrentMeasurement=yes  SetLabelI=off  LabelI=Igri  Ipu=off  Pbase=100e6  Vbase=500e3  OutputType=Complex  PhasorSimulation=off  PSBequivalent=0
  A : PMIOPort  Side=Left
  B : PMIOPort  Port=2  Side=Left
  a : PMIOPort  Port=3  Side=Right
  b : PMIOPort  Port=4  Side=Right
  C : PMIOPort  Port=5  Side=Left
  c : PMIOPort  Port=6  Side=Right
  tag scope: Igri=scoped, Ugri=scoped
  wires:
  GRI1/1 -> [Ugri]
  GRI1/2 -> [Igri]
  connections:
  GRI1/LConn3 -- C/RConn1
  GRI1/LConn2 -- B/RConn1
  GRI1/RConn3 -- c/RConn1
  GRI1/RConn2 -- b/RConn1
  GRI1/LConn1 -- A/RConn1
  GRI1/RConn1 -- a/RConn1

== system Microgrid_transition_model_111821_ben/Stab1/AllStringInverters/BESS Inverter ==
  ctrl : Inport
  Controlled Voltage Source : powerlib/Electrical Sources/Controlled Voltage Source  Initialize=on  Source_Type=AC  Amplitude=0  Phase=0  Frequency=0  Measurements=None
  Controlled Voltage Source1 : powerlib/Electrical Sources/Controlled Voltage Source  Initialize=on  Source_Type=AC  Amplitude=0  Phase=0  Frequency=0  Measurements=None
  Controlled Voltage Source2 : powerlib/Electrical Sources/Controlled Voltage Source  Initialize=on  Source_Type=AC  Amplitude=0  Phase=0  Frequency=0  Measurements=None
  Demux : Demux  Outputs=3
  A : PMIOPort  Side=Right
  N : PMIOPort  Port=2  Side=Left
  B : PMIOPort  Port=3  Side=Right
  C : PMIOPort  Port=4  Side=Right
  wires:
  ctrl/1 -> Demux/1
  Demux/3 -> Controlled Voltage Source2/1
  Demux/2 -> Controlled Voltage Source1/1
  Demux/1 -> Controlled Voltage Source/1
  connections:
  Controlled Voltage Source2/RConn1 -- C/RConn1
  Controlled Voltage Source1/RConn1 -- B/RConn1
  N/RConn1 -- Controlled Voltage Source1/LConn1 -- Controlled Voltage Source/LConn1 -- Controlled Voltage Source2/LConn1
  A/RConn1 -- Controlled Voltage Source/RConn1

== system Microgrid_transition_model_111821_ben/Stab1/AllStringInverters/PV_Control ==
  Uabc : Inport
  Uabc_inv : Inport  Port=2
  Iabc : Inport  Port=3
  CB_status : Inport  Port=4
  Control : Inport  Port=5
  Bus Creator1 : BusCreator  Inputs=2
  Bus Creator5 : BusCreator  Inputs=1
  Bus Selector : BusSelector  OutputSignals=p_ref,q_ref,f_ref,v_ref,GF_mode
  InvControl : Subsystem  mask{Ts=Ts_Control, Unpp=600, Pn=430e3}
      mask prompts: Ts "Control sample time [s]"; Unpp "Nominal AC voltage [Vpp]"; Pn "Nominal Power [W]"
      mask init:
      | Unom = Unpp / sqrt(3);
      | Inom = Pn/3/Unom;
  Rate Transition{,1..2,4..7,9..10} (9 alike) : RateTransition  Integrity=off  OutPortSampleTime=Ts_Control
  Rate Transition3 : RateTransition  OutPortSampleTime=Ts
  Rate Transition8 : RateTransition  OutPortSampleTime=Ts
  Step : Step  Time=3  SampleTime=0
  Step1 : Step  Time=6.4  SampleTime=0
  Sum : Sum  Inputs=|++
  CtrlOut : Outport
  wires:
  Step1/1 -> Sum/2
  Step/1 -> Sum/1
  Rate Transition4/1 -> InvControl/5(pref)
  Iabc/1 -> Rate Transition1/1
  Rate Transition2/1 -> InvControl/4(cb_stat)
  Rate Transition1/1 -> InvControl/3(Iabc)
  Rate Transition/1 -> InvControl/1(Uabc)
  Rate Transition8/1 -> Bus Creator5/1  "Close"
  Sum/1 -> Rate Transition8/1
  InvControl/1(Uabc_ref) -> Rate Transition3/1
  Rate Transition3/1 -> Bus Creator1/1  "Uabc"
  Uabc/1 -> Rate Transition/1
  CB_status/1 -> Rate Transition2/1
  Bus Creator5/1 -> Bus Creator1/2  "ToCB"
  Bus Creator1/1 -> CtrlOut/1
  Bus Selector/1 -> Rate Transition4/1  "<p_ref>"
  Bus Selector/2 -> Rate Transition5/1  "<q_ref>"
  Bus Selector/3 -> Rate Transition6/1  "<f_ref>"
  Bus Selector/4 -> Rate Transition7/1  "<v_ref>"
  Bus Selector/5 -> Rate Transition9/1  "<GF_mode>"
  Rate Transition9/1 -> InvControl/9(GF_mode_en)
  Rate Transition7/1 -> InvControl/8(vref)
  Rate Transition5/1 -> InvControl/6(qref)
  Rate Transition6/1 -> InvControl/7(fref)
  Control/1 -> Bus Selector/1
  Uabc_inv/1 -> Rate Transition10/1
  Rate Transition10/1 -> InvControl/2(Uabc_inv)
